simulink model "prob4"  (R2020b)
settings: Solver=VariableStepAuto  StartTime=0.0  StopTime=3  RelTol=1e-3
settings Model: Creator=diego  LastModifiedBy=diego

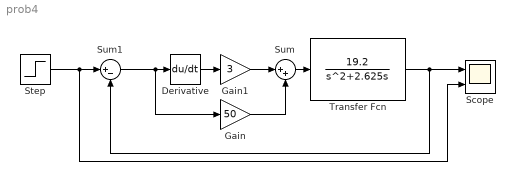
== system prob4 ==
  Derivative : Derivative
  Gain : Gain  Gain=50
  Gain1 : Gain  Gain=3
  Scope : Scope  NumInputPorts=2
  Step : Step  SampleTime=0
  Sum : Sum  Inputs=|++
  Sum1 : Sum  Inputs=|+-
  Transfer Fcn : TransferFcn  Numerator=[19.2]  Denominator=[1 2.625 0]
  wires:
  Gain/1 -> Sum/2
  Sum/1 -> Transfer Fcn/1
  Transfer Fcn/1 -> Sum1/2, Scope/1
  Step/1 -> Scope/2, Sum1/1
  Sum1/1 -> Gain/1, Derivative/1
  Derivative/1 -> Gain1/1
  Gain1/1 -> Sum/1
